simulink subsystem "Day1_Scenario_1"  (R2024a)
settings: Solver=VariableStepAuto  StartTime=0.0  StopTime=10.0  RelTol=1e-3
libraries: CarMaker4SL x1
settings Model: Creator=junhyung.cha  LastModifiedBy=User

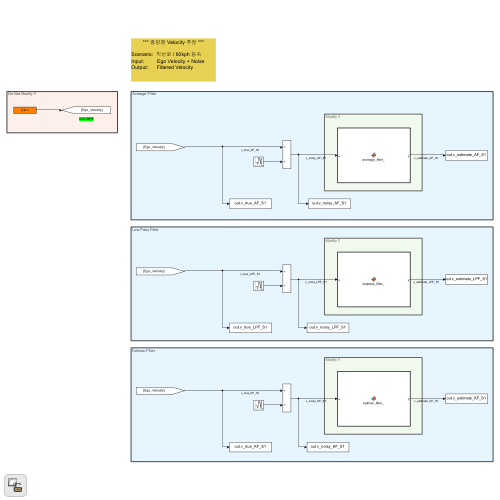
[thumbnail: Simulink's stored preview of the top-level diagram]
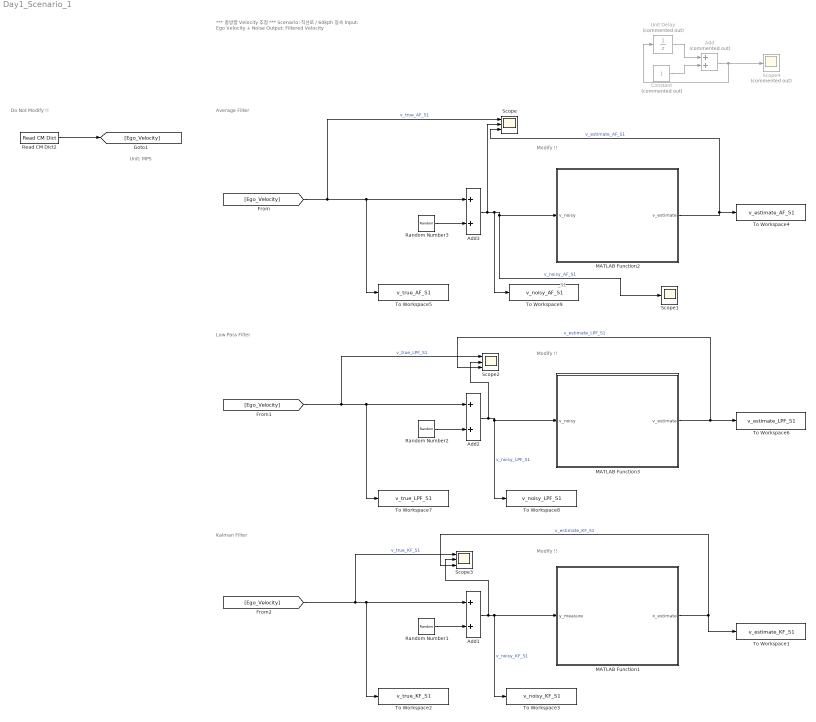
== system Day1_Scenario_1 ==
  note: _S1
  note: Modify !!
  note: Modify !!
  note: Modify !!
  note: Average Filter
  note: Low Pass Filter
  note: Kalman Filter
  note: *** 종방향 Velocity 추정 ***
      |
      | Scenario: 직선로 / 60kph 등속
      | Input: Ego Velocity + Noise
      | Output: Filtered Velocity
  note: Do Not Modify !!
  note: Unit: MPS
  Add : Sum  Commented=on
  Add1 : Sum
  Add2 : Sum
  Add3 : Sum
  Constant : Constant  Commented=on  SampleTime=-1
  MATLAB Function1 : MATLAB Function  TreatAsAtomicUnit=on
  MATLAB Function2 : MATLAB Function  TreatAsAtomicUnit=on
  MATLAB Function3 : MATLAB Function  TreatAsAtomicUnit=on
  Random Number1 : RandomNumber
  Random Number2 : RandomNumber
  Random Number3 : RandomNumber
  Read CM Dict2 : CarMaker4SL/Read CM Dict  xname=Car.v  xsync=off  xstime=Inherited
  Scope : Scope  NumInputPorts=3
  Scope1 : Scope
  Scope2 : Scope  NumInputPorts=3
  Scope3 : Scope  NumInputPorts=3
  Scope4 : Scope  Commented=on
  To Workspace1 : ToWorkspace  VariableName=v_estimate_KF_S1  SaveFormat=Timeseries  SampleTime=-1
  To Workspace2 : ToWorkspace  VariableName=v_true_KF_S1  SaveFormat=Timeseries  SampleTime=-1
  To Workspace3 : ToWorkspace  VariableName=v_noisy_KF_S1  SaveFormat=Timeseries  SampleTime=-1
  To Workspace4 : ToWorkspace  VariableName=v_estimate_AF_S1  SaveFormat=Timeseries  SampleTime=-1
  To Workspace5 : ToWorkspace  VariableName=v_true_AF_S1  SaveFormat=Timeseries  SampleTime=-1
  To Workspace6 : ToWorkspace  VariableName=v_estimate_LPF_S1  SaveFormat=Timeseries  SampleTime=-1
  To Workspace7 : ToWorkspace  VariableName=v_true_LPF_S1  SaveFormat=Timeseries  SampleTime=-1
  To Workspace8 : ToWorkspace  VariableName=v_noisy_LPF_S1  SaveFormat=Timeseries  SampleTime=-1
  To Workspace9 : ToWorkspace  VariableName=v_noisy_AF_S1  SaveFormat=Timeseries  SampleTime=-1
  Unit Delay : UnitDelay  Commented=on  SampleTime=-1  HasFrameUpgradeWarning=on
  wires:
  Random Number2/1 -> Add2/2
  [Ego_Velocity] -> Add2/1, To Workspace7/1, Scope2/1  "v_true_LPF_S1"
  Add2/1 -> MATLAB Function3/1(v_noisy), To Workspace8/1, Scope2/2  "v_noisy_LPF_S1"
  MATLAB Function3/1(v_estimate) -> To Workspace6/1, Scope2/3  "v_estimate_LPF_S1"
  [Ego_Velocity] -> Add1/1, To Workspace2/1, Scope3/1  "v_true_KF_S1"
  MATLAB Function1/1(x_estimate) -> Scope3/3, To Workspace1/1  "v_estimate_KF_S1"
  Random Number1/1 -> Add1/2
  Add1/1 -> MATLAB Function1/1(y_measure), To Workspace3/1, Scope3/2  "v_noisy_KF_S1"
  MATLAB Function2/1(v_estimate) -> To Workspace4/1, Scope/3  "v_estimate_AF_S1"
  Random Number3/1 -> Add3/2
  [Ego_Velocity] -> Add3/1, To Workspace5/1, Scope/1  "v_true_AF_S1"
  Add3/1 -> MATLAB Function2/1(v_noisy), Scope1/1, To Workspace9/1, Scope/2  "v_noisy_AF_S1"
  Read CM Dict2/1 -> [Ego_Velocity]
  Unit Delay/1 -> Add/1
  Constant/1 -> Add/2
  Add/1 -> Scope4/1, Unit Delay/1

== matlab function Day1_Scenario_1/MATLAB Function1 ==
  settings: updateMethod=DISCRETE  sampleTime=0.05
  data: y_measure input; x_estimate output
function x_estimate = kalman_filter_step(y_measure)
% y_measure: 현재 측정값 (v_noisy_KF_S1)
% x_estimate: 필터 추정 출력

persistent x_est P_est A B C Q R dt

% 고정된 dt 값 (시간 간격)
if isempty(dt)
    dt = 0.1;  % 샘플링 시간 (예: 0.1초)
end

% 필터 파라미터
if isempty(x_est)
    % 초기화 (필터의 초기 상태 및 공분산)
    A = [1.0, dt; 0.0, 1.0];  % 상태 전이 행렬 (A * dt)
    B = [0.0; dt];             % 입력 제어 행렬 (여기서는 입력 없음)
    C = [1.0, 0.0];            % 측정 행렬
    Q = [0.01, 0; 0, 0.01];    % 모델 노이즈 공분산
    R = 1.0;                   % 측정 노이즈 공분산
    x_est = [y_measure; 0.0];  % 초기 상태 추정 (위치, 속도)
    P_est = [10.0, 0.0; 0.0, 10.0];  % 초기 공분산
end

% Prediction (예측)
A_dt = A * dt + eye(size(A));  % 상태 전이 행렬 업데이트 (Adt + I)
x_pred = A_dt * x_est;         % 예측된 상태
P_pred = A_dt * P_est * A_dt' + Q;  % 공분산 예측

% Kalman Gain 계산
S = C * P_pred * C' + R;  % S 계산
K = P_pred * C' / S;      % 칼만 이득 계산

% Update (업데이트)
y_error = y_measure - C * x_pred;  % 측정 오차
x_est = x_pred + K * y_error;      % 상태 추정 업데이트
P_est = (eye(size(P_est)) - K * C) * P_pred;  % 공분산 업데이트

% 출력
x_estimate = x_est;  % 최종 상태 추정값 출력
end

== matlab function Day1_Scenario_1/MATLAB Function2 ==
  settings: updateMethod=DISCRETE  sampleTime=0.05
  data: v_noisy input; v_estimate output
function v_estimate = average_filter_step(v_noisy)
% Simulink에서 상태 유지형 평균 필터
% 입력: v_noisy (현재 샘플)
% 출력: v_estimate (필터 출력)

persistent v_prev_est k
if isempty(v_prev_est)
    v_prev_est = v_noisy;
    k = 1;
    v_estimate = v_noisy;
    return;
end

k = k + 1;
v_estimate = ((k - 1)/k) * v_prev_est + (1/k) * v_noisy;

% 상태 저장
v_prev_est = v_estimate;


% function [y, i_out] = average_filter_(u)
% 
% persistent i
% if isempty(i)
%     i = 0;
% end
% 
% i = i+1;
% i_out = i;
% 
% if i> 10
%     i = 0;
% end
% 
% y = 0;
% end

== matlab function Day1_Scenario_1/MATLAB Function3 ==
  settings: updateMethod=DISCRETE  sampleTime=0.05
  data: v_noisy input; v_estimate output
function v_estimate = low_pass_filter_step(v_noisy)
% v_estimate: 필터 출력
% v_noisy: 노이즈가 있는 입력
% 내부 상태 유지 위해 persistent 사용

persistent v_est_prev
alpha = 0.9;

if isempty(v_est_prev)
    v_est_prev = v_noisy;
end

% 필터 식
v_estimate = alpha * v_est_prev + (1 - alpha) * v_noisy;

% 상태 업데이트
v_est_prev = v_estimate;
